simulink model "demoAUVdepthPIDcontrol_longitudinal"  (R2023a)
settings: Solver=VariableStepAuto  StartTime=0.0  StopTime=400  RelTol=1e-3
libraries: slpidlib x1, mssSimulink x1
settings Model: Creator=23147  LastModifiedBy=23147
settings DataIOCC: ExternalInput=[x_target, z_target]

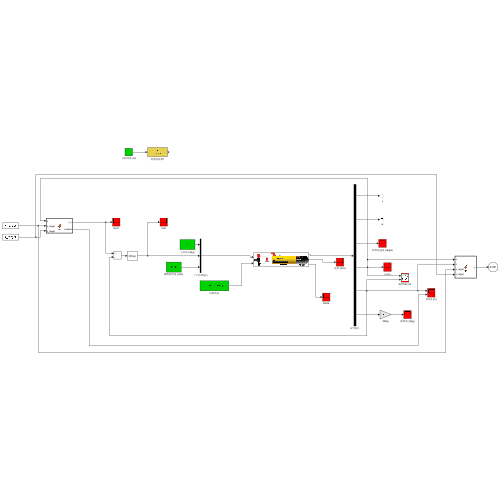
[thumbnail: Simulink's stored preview of the top-level diagram]
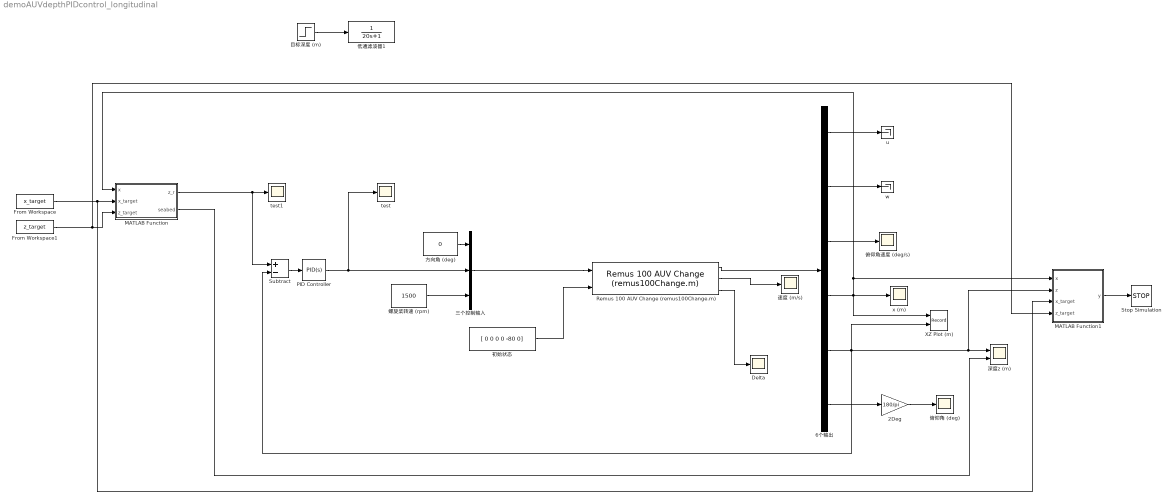
== system demoAUVdepthPIDcontrol_longitudinal ==
  2Deg : Gain  Gain=180/pi
  6个输出 : Demux  Outputs=6
  Delta : Scope
  From Workspace : FromWorkspace  VariableName=x_target
  From Workspace1 : FromWorkspace  VariableName=z_target
  MATLAB Function : MATLAB Function  TreatAsAtomicUnit=on
  MATLAB Function1 : MATLAB Function  TreatAsAtomicUnit=on
  PID Controller : slpidlib/PID Controller  Controller=PID  Form=Parallel  TimeDomain=Continuous-time  UseExternalTs=off  SampleTime=-1  IntegratorMethod=Forward Euler  FilterMethod=Forward Euler  ControllerParametersSource=internal  P=100  I=0.01  UseKiTs=off  D=500  N=100  UseFilter=on  TunerSelectOption=Transfer Function Based (PID Tuner App)  InitialConditionSource=internal  InitialConditionForIntegrator=0  InitialConditionForFilter=0  DifferentiatorICPrevScaledInput=0  ExternalReset=none  TrackingMode=off  Kt=1  LimitOutput=off  SatLimitsSource=internal  UpperSaturationLimit=inf  LowerSaturationLimit=-inf  LinearizeAsGain=on  AntiWindupMode=none  Kb=1  LimitIntegrator=off  UpperIntegratorSaturationLimit=inf  LowerIntegratorSaturationLimit=-inf  POutMin=[]  POutMax=[]  IOutMin=[]  IOutMax=[]  DOutMin=[]  DOutMax=[]  NOutMin=[]  NOutMax=[]  SumOutMin=[]  SumOutMax=[]  SaturationOutMin=[]  SaturationOutMax=[]  PParamMin=[]  PParamMax=[]  IParamMin=[]  IParamMax=[]  DParamMin=[]  DParamMax=[]  NParamMin=[]  NParamMax=[]  KbParamMin=[]  KbParamMax=[]  KtParamMin=[]  KtParamMax=[]  KbOutMin=[]  KbOutMax=[]  KtOutMin=[]  KtOutMax=[]  IntegratorOutMin=[]  IntegratorOutMax=[]  FilterOutMin=[]  FilterOutMax=[]  SumI1OutMin=[]  SumI1OutMax=[]  SumI2OutMin=[]  SumI2OutMax=[]  SumI3OutMin=[]  SumI3OutMax=[]  SumI4OutMin=[]  SumI4OutMax=[]  SumDOutMin=[]  SumDOutMax=[]  DifferentiatorOutMin=[]  DifferentiatorOutMax=[]  FilterDiffOutCoefMin=[]  FilterDiffOutCoefMax=[]  ReciprocalOutMin=[]  ReciprocalOutMax=[]  SumDenOutMin=[]  SumDenOutMax=[]  SumNumOutMin=[]  SumNumOutMax=[]  DivideOutMin=[]  DivideOutMax=[]  UdiffTsProdOutMin=[]  UdiffTsProdOutMax=[]  NTsProdOutMin=[]  NTsProdOutMax=[]  UintegralTsProdOutMin=[]  UintegralTsProdOutMax=[]  UngainTsProdOutMin=[]  UngainTsProdOutMax=[]  ClampingZeroOutDataTypeStr=Inherit: Inherit via back propagation  ClampingZeroOutMin=[]  ClampingZeroOutMax=[]  FilterDenConstantOutDataTypeStr=Inherit: Inherit via back propagation  FilterDenConstantOutMin=[]  FilterDenConstantOutMax=[]  PCopyOutDataTypeStr=Inherit: Inherit via back propagation  PCopyOutMin=[]  PCopyOutMax=[]  NCopyOutDataTypeStr=Inherit: Inherit via back propagation  NCopyOutMin=[]  NCopyOutMax=[]  IntegratorContinuousStateAttributes=''  IntegratorStateMustResolveToSignalObject=off  IntegratorRTWStateStorageClass=Auto  FilterContinuousStateAttributes=''  FilterStateMustResolveToSignalObject=off  FilterRTWStateStorageClass=Auto  ParallelPVariant=InternalParameters  IdealPVariant=Disabled  IVariant=InternalParameters  DVariant=InternalParameters  IntegratorVariant=Continuous  SatVariant=Disabled  AWVariant=Passthrough  PCopyVariant=Disabled  TRVariant=Disabled  FdbkBlocksVariant=Forward  IdealPFdbkVariant=Disabled  SatFdbkVariant=Disabled  DerivativeFilterVariant=ContFilter  NVariant=InternalParameters  NCopyVariant=Disabled  FilterICVariant=InternalICsFilter  IntegratorICVariant=InternalICs  ExternalResetVariant=Disabled  TRSumVariant=Passthrough  SumFdbkVariant=Disabled  SumVariant=Sum_PID  TsampFilterVariant=InternalTs  TsampNgainVariant=Passthrough  TsampIntegralVariant=Disabled_SignalSpec  ExternalSaturationOutDataTypeStr=Inherit: Same as second input
  Remus 100 AUV Change (remus100Change.m) : mssSimulink/Marine craft models/Remus 100 AUV Change (remus100Change.m)  SystemSampleTime=-1  VariantActivationTime=update diagram  Latency=0  AutoFrameSizeCalculation=off
  Stop Simulation : Stop
  Subtract : Sum  Inputs=+-
  XZ Plot (m) : Record  FileSettingsInternal="{\"entries\":[{\"content\":{\"excelSettings\":{\"content\":{},\"type\":\"Streamout.ExcelSettings\"}},\"type\":\"Streamout.FileSettingStorage\",\"uuid\":\"\"}],\"packageUris\":[\"http:\\/\\/schema.mathworks.com\\/mf0\\/streamout_blocks\\/R2020a\"],\"version\":\"1.0\"}"  Layout=[1 1]  SignalsInternal="{\"entries\":[{\"content\":{\"signals\":[{\"content\":{\"blockPath\":[],\"dimensions\":[1,1],\"domain\":\"\",\"lineColor\":\"#77ac30\",\"plots\":[1],\"port\":1,\"sid\":[\"\"],\"signalID\":19,\"signalName\":\"6个输出:4\"},\"type\":\"RecordBlkView.Signal\",\"uuid\":\"\"},{\"content\":{\"blockPath\":[],\"dimensions\":[1,1],\"domain\":\"\",\"lineColor\":\"#4dbeee\",\"plots\":[1],\"port\":2,\"sid\":[\"\"],\"signalID\":23,\"signalName\":\"6个输出:5\"},\"type\":\"RecordBlkView.Signal\",\"uuid\":\"\"}]},\"type\":\"RecordBlkView.InputSignals\",\"uuid\":\"\"}],\"packageUris\":[\"http:\\/\\/schema.mathworks.com\\/mf0\\/streamout_blocks\\/R2020a\"],\"version\":\"1.0\"}"  VisualizationBindings="{\"xyplotplugin\":{\"info\":[{\"series\":[{\"bindingParametersList\":[{\"parameter\":\"Y-Axis\",\"signalID\":23,\"signalName\":\"6个输出:5\"}],\"seriesID\":771},{\"bindingParametersList\":[{\"parameter\":\"Y-Axis\",\"signalID\":23,\"signalName\":\"6个输出:5\"},{\"parameter\":\"X-Axis\",\"signalID\":19,\"signalName\":\"6个输出:4\"}],\"seriesID\":37341}],\"subplotID\":1}]}}"  CompatibilityTag=XY  st=-1
  test : Scope
  test1 : Scope
  u : Terminator
  w : Terminator
  x (m) : Scope
  三个控制输入 : Mux  Inputs=[1 1 1]
  低通滤波器1 : TransferFcn  Denominator=[20 1]
  俯仰角 (deg) : Scope
  俯仰角速度 (deg/s) : Scope
  初始状态 : Constant  Value=[ 0 0 0 0 -80 0]
  方向角 (deg) : Constant  Value=0
  深度z (m) : Scope  NumInputPorts=2
  目标深度 (m) : Step  Time=200  Before=-100  After=-150  SampleTime=0
  螺旋桨转速 (rpm) : Constant  Value=1500
  速度 (m/s) : Scope
  wires:
  初始状态/1 -> Remus 100 AUV Change (remus100Change.m)/2
  三个控制输入/1 -> Remus 100 AUV Change (remus100Change.m)/1
  螺旋桨转速 (rpm)/1 -> 三个控制输入/3
  方向角 (deg)/1 -> 三个控制输入/1
  Remus 100 AUV Change (remus100Change.m)/2 -> 速度 (m/s)/1
  Remus 100 AUV Change (remus100Change.m)/1 -> 6个输出/1
  6个输出/1 -> u/1
  6个输出/2 -> w/1
  2Deg/1 -> 俯仰角 (deg)/1
  MATLAB Function/1(z_r) -> Subtract/1, test1/1
  Subtract/1 -> PID Controller/1
  PID Controller/1 -> test/1, 三个控制输入/2
  6个输出/3 -> 俯仰角速度 (deg/s)/1
  6个输出/4 -> MATLAB Function/1(x), MATLAB Function1/1(x), XZ Plot (m)/1, x (m)/1
  6个输出/5 -> 深度z (m)/1, MATLAB Function1/2(z), XZ Plot (m)/2, Subtract/2
  6个输出/6 -> 2Deg/1
  From Workspace/1 -> MATLAB Function1/3(x_target), MATLAB Function/2(x_target)
  From Workspace1/1 -> MATLAB Function1/4(z_target), MATLAB Function/3(z_target)
  MATLAB Function/2(seabed) -> 深度z (m)/2
  MATLAB Function1/1(y) -> Stop Simulation/1
  目标深度 (m)/1 -> 低通滤波器1/1
  Remus 100 AUV Change (remus100Change.m)/3 -> Delta/1

== matlab function demoAUVdepthPIDcontrol_longitudinal/MATLAB Function1 ==
  data: x input; y output; z input; x_target input; z_target input
function y = fcn(x, z, x_target, z_target)
z_r = interp1(x_target,z_target,x,'spline');
if z_r > z
    y = 0;
else
    y = 0;
end

== matlab function demoAUVdepthPIDcontrol_longitudinal/MATLAB Function ==
  data: x input; z_r output; x_target input; z_target input; seabed output
function [z_r, seabed] = fcn(x, x_target, z_target)
%x_target = 0:0.01:1000;
%z_target=10*sin(0.05*x_target)-100;
seabed = interp1(x_target,z_target,x,'spline');
z_r = seabed + 10;
